simulink subsystem "GroundSystem"  (R2019b)
settings: Solver=VariableStepAuto  StartTime=0.0  StopTime=10.0  RelTol=1e-3
undefined symbols (not defined in the file): constr, Lbooth, loiterStates, params
libraries: simulink x4
settings Model: Creator=dylaneijkelhof  LastModifiedBy=dylaneijkelhof

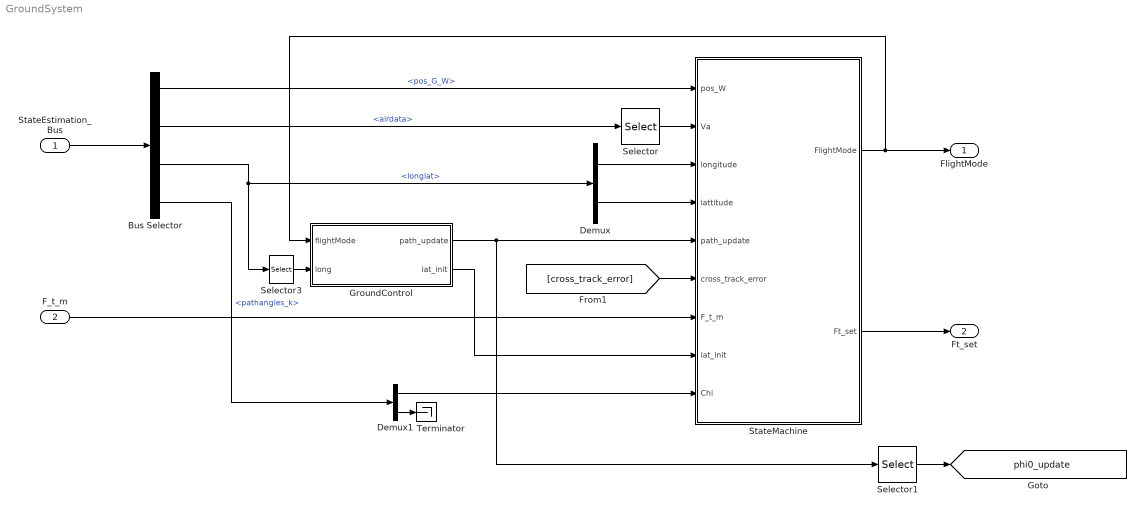
== system GroundSystem ==
  StateEstimation_Bus : Inport
  F_t_m : Inport  Port=2
  Bus Selector : BusSelector  OutputSignals=pos_G_W,airdata,longlat,pathangles_k
  Demux : Demux  Outputs=2
  Demux1 : Demux  Outputs=2
  GroundControl : Subsystem
  Selector : Selector  InputPortWidth=3  IndexOptions=Index vector (dialog)  Indices=1  OutputSizes=1
  Selector1 : Selector  InputPortWidth=3  IndexOptions=Index vector (dialog)  Indices=1  OutputSizes=1
  Selector3 : Selector  InputPortWidth=2  IndexOptions=Index vector (dialog)  Indices=1  OutputSizes=1
  StateMachine : Subsystem
  Terminator : Terminator
  FlightMode : Outport  VectorParamsAs1DForOutWhenUnconnected=off
  Ft_set : Outport  Port=2  VectorParamsAs1DForOutWhenUnconnected=off
  tag scope: phi0_update=global
  wires:
  Selector/1 -> StateMachine/2(Va)
  Bus Selector/2 -> Selector/1  "<airdata>"
  Bus Selector/1 -> StateMachine/1(pos_W)  "<pos_G_W>"
  StateEstimation_Bus/1 -> Bus Selector/1
  Demux/1 -> StateMachine/3(longitude)
  StateMachine/2(Ft_set) -> Ft_set/1
  Demux/2 -> StateMachine/4(lattitude)
  [cross_track_error] -> StateMachine/6(cross_track_error)
  F_t_m/1 -> StateMachine/7(F_t_m)
  Bus Selector/3 -> Demux/1, Selector3/1  "<longlat>"
  StateMachine/1(FlightMode) -> GroundControl/1(flightMode), FlightMode/1
  Selector1/1 -> [phi0_update]
  GroundControl/1(path_update) -> StateMachine/5(path_update), Selector1/1
  Selector3/1 -> GroundControl/2(long)
  GroundControl/2(lat_init) -> StateMachine/8(lat_init)
  Bus Selector/4 -> Demux1/1  "<pathangles_k>"
  Demux1/2 -> Terminator/1
  Demux1/1 -> StateMachine/9(Chi)

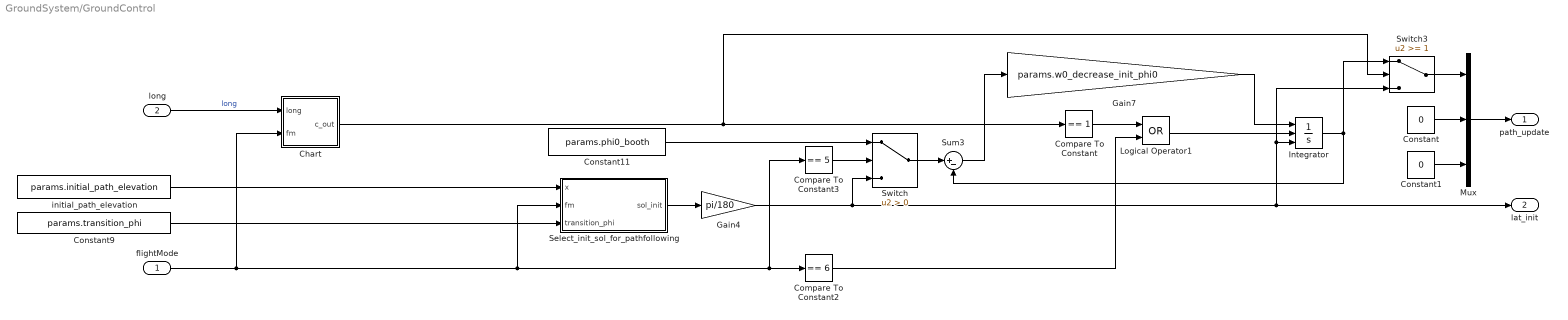
== system GroundSystem/GroundControl ==
  flightMode : Inport
  long : Inport  Port=2
  Chart : Stateflow chart  TreatAsAtomicUnit=on
  Compare To Constant : simulink/Logic and Bit Operations/Compare To Constant  relop===  const=1  OutDataTypeStr=boolean
  Compare To Constant2 : simulink/Logic and Bit Operations/Compare To Constant  relop===  const=6  OutDataTypeStr=boolean
  Compare To Constant3 : simulink/Logic and Bit Operations/Compare To Constant  relop===  const=5  OutDataTypeStr=boolean
  Constant : Constant  Value=0
  Constant1 : Constant  Value=0
  Constant11 : Constant  Value=params.phi0_booth
  Constant9 : Constant  Value=params.transition_phi
  Gain4 : Gain  Gain=pi/180
  Gain7 : Gain  Gain=params.w0_decrease_init_phi0
  Integrator : Integrator  ExternalReset=rising  InitialConditionSource=external
  Logical Operator1 : Logic  Operator=OR  AllPortsSameDT=off  OutDataTypeStr=boolean
  Mux : Mux  Inputs=3
  Select_init_sol_for_pathfollowing : Stateflow chart  TreatAsAtomicUnit=on
  Sum3 : Sum  Inputs=|+-
  Switch : Switch  Criteria=u2 > Threshold
  Switch3 : Switch  Threshold=1
  initial_path_elevation : Constant  Value=params.initial_path_elevation
  path_update : Outport  PortDimensions=[3,1]  VectorParamsAs1DForOutWhenUnconnected=off
  lat_init : Outport  Port=2  VectorParamsAs1DForOutWhenUnconnected=off
  wires:
  Constant11/1 -> Switch/1
  Constant9/1 -> Select_init_sol_for_pathfollowing/3(transition_phi)
  Switch3/1 -> Mux/1
  Gain7/1 -> Integrator/1
  Logical Operator1/1 -> Integrator/2
  Compare To Constant/1 -> Logical Operator1/1
  Integrator/1 -> Switch3/1, Sum3/2
  Gain4/1 -> Switch/3, lat_init/1, Integrator/3, Switch3/3
  Chart/1(c_out) -> Compare To Constant/1, Switch3/2
  long/1 -> Chart/1(long)  "long"
  initial_path_elevation/1 -> Select_init_sol_for_pathfollowing/1(x)
  Compare To Constant3/1 -> Switch/2
  Switch/1 -> Sum3/1
  Compare To Constant2/1 -> Logical Operator1/2
  flightMode/1 -> Chart/2(fm), Compare To Constant2/1, Compare To Constant3/1, Select_init_sol_for_pathfollowing/2(fm)
  Select_init_sol_for_pathfollowing/1(sol_init) -> Gain4/1
  Sum3/1 -> Gain7/1
  Mux/1 -> path_update/1
  Constant/1 -> Mux/2
  Constant1/1 -> Mux/3

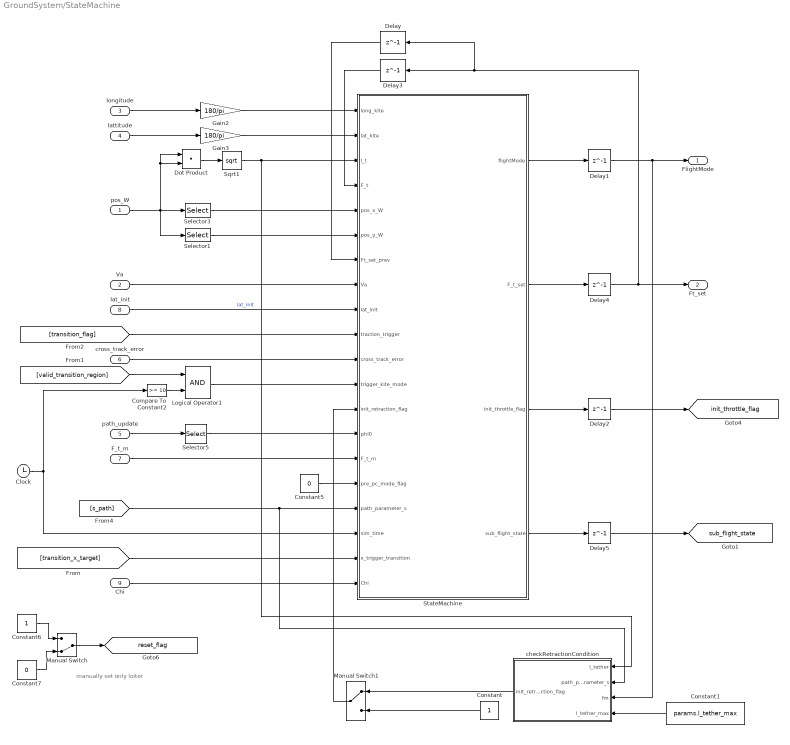
== system GroundSystem/StateMachine ==
  note: manually set only loiter
  pos_W : Inport
  Va : Inport  Port=2
  longitude : Inport  Port=3
  lattitude : Inport  Port=4
  path_update : Inport  Port=5
  cross_track_error : Inport  Port=6
  F_t_m : Inport  Port=7
  lat_init : Inport  Port=8
  Chi : Inport  Port=9
  Clock : Clock
  Compare To Constant2 : simulink/Logic and Bit Operations/Compare To Constant  relop=>=  const=10  OutDataTypeStr=boolean
  Constant : Constant
  Constant1 : Constant  Value=params.l_tether_max
  Constant5 : Constant  Value=0
  Constant6 : Constant
  Constant7 : Constant  Value=0
  Delay : Delay  DelayLength=1  InitialCondition=100
  Delay1 : Delay  DelayLength=1
  Delay2 : Delay  DelayLength=1  InitialCondition=1
  Delay3 : Delay  DelayLength=1  InitialCondition=100
  Delay4 : Delay  DelayLength=1
  Delay5 : Delay  DelayLength=1  InitialCondition=1
  Dot Product : DotProduct  InputSameDT=on  OutDataTypeStr=Inherit: Inherit via internal rule
  Gain2 : Gain  Gain=180/pi
  Gain3 : Gain  Gain=180/pi
  Logical Operator1 : Logic  AllPortsSameDT=off  OutDataTypeStr=boolean
  Manual Switch : ManualSwitch  CurrentSetting=0
  Manual Switch1 : ManualSwitch
  Selector1 : Selector  InputPortWidth=3  IndexOptions=Index vector (dialog)  Indices=2  OutputSizes=1
  Selector3 : Selector  InputPortWidth=3  IndexOptions=Index vector (dialog)  Indices=1  OutputSizes=1
  Selector5 : Selector  InputPortWidth=3  IndexOptions=Index vector (dialog)  Indices=1  OutputSizes=1
  Sqrt1 : Sqrt  SaturateOnIntegerOverflow=on
  StateMachine : Stateflow chart  TreatAsAtomicUnit=on  mask{F_T_traction_set=params.F_t_traction_set, F_set_retraction=params.F_t_retraction_set*params.F_t_traction_set, l_t_min=params.l_tether_min, l_t_max=params.l_tether_max, a_booth=params.a_booth, b_booth=params.b_booth, lat_trans=0, alpha2=params.ft_smooth_2, crosstrackerror_condition=params.crosstrackerror_condition, Vamin=constr.Va_min, Ft_set_loiter=loiterStates.Ft_set_loiter}
      mask prompts: F_T_traction_set "Traction force"; F_set_retraction "Retraction force"; l_t_min "Min. tether length"; l_t_max "Max. tether length"; a_booth "abooth"; b_booth "bbooth"; alpha2 "interpolation factor retrac 2 trac"
  checkRetractionCondition : Stateflow chart  TreatAsAtomicUnit=on
  FlightMode : Outport  VectorParamsAs1DForOutWhenUnconnected=off
  Ft_set : Outport  Port=2  VectorParamsAs1DForOutWhenUnconnected=off
  tag scope: init_throttle_flag=global, reset_flag=global, sub_flight_state=global
  wires:
  Chi/1 -> StateMachine/20(Chi)
  [transition_x_target] -> StateMachine/19(x_trigger_transition)
  Delay5/1 -> [sub_flight_state]
  Constant/1 -> Manual Switch1/2
  checkRetractionCondition/1(init_retraction_flag) -> Manual Switch1/1
  lat_init/1 -> StateMachine/9(lat_init)  "lat_init"
  [s_path] -> StateMachine/17(path_parameter_s), checkRetractionCondition/2(path_parameter_s)
  Clock/1 -> StateMachine/18(sim_time), Compare To Constant2/1
  Manual Switch/1 -> [reset_flag]
  Constant7/1 -> Manual Switch/2
  Constant6/1 -> Manual Switch/1
  [transition_flag] -> StateMachine/10(traction_trigger)
  Constant5/1 -> StateMachine/16(pre_pc_mode_flag)
  F_t_m/1 -> StateMachine/15(F_t_m)
  StateMachine/4(sub_flight_state) -> Delay5/1
  Delay4/1 -> Delay3/1, Delay/1, Ft_set/1
  Sqrt1/1 -> StateMachine/3(l_t), checkRetractionCondition/1(l_tether)
  Gain3/1 -> StateMachine/2(lat_kite)
  path_update/1 -> Selector5/1
  Selector5/1 -> StateMachine/14(phi0)
  Delay3/1 -> StateMachine/4(F_t)
  StateMachine/1(flightMode) -> Delay1/1
  Gain2/1 -> StateMachine/1(long_kite)
  pos_W/1 -> Selector3/1, Selector1/1, Dot Product/2, Dot Product/1
  Selector3/1 -> StateMachine/5(pos_x_W)
  Dot Product/1 -> Sqrt1/1
  Delay/1 -> StateMachine/7(Ft_set_prev)
  Selector1/1 -> StateMachine/6(pos_y_W)
  cross_track_error/1 -> StateMachine/11(cross_track_error)
  Logical Operator1/1 -> StateMachine/12(trigger_kite_mode)
  Compare To Constant2/1 -> Logical Operator1/2
  [valid_transition_region] -> Logical Operator1/1
  Delay1/1 -> checkRetractionCondition/3(fm), FlightMode/1
  StateMachine/3(init_throttle_flag) -> Delay2/1
  Delay2/1 -> [init_throttle_flag]
  longitude/1 -> Gain2/1
  lattitude/1 -> Gain3/1
  StateMachine/2(F_t_set) -> Delay4/1
  Va/1 -> StateMachine/8(Va)
  Constant1/1 -> checkRetractionCondition/4(l_tether_max)
  Manual Switch1/1 -> StateMachine/13(init_retraction_flag)

== stateflow chart GroundSystem/StateMachine/StateMachine ==
  state loiter
    entry: flightMode = 1;
    during: F_t_set = Ft_set_loiter;
    entry: init_throttle_flag = 1;
    entry: sub_flight_state = 1;
  state Traction4 % slowly increase tether force
    entry: flightMode=5;
    during: F_t_set = calcSetpoint(alpha2,Ft_set_prev,Ft_set_loiter);
    exit: init_throttle_flag = 1;
    entry: sub_flight_state = 2;
  note: F_t_m>F_set_retraction
  note: pos_x_W<x_trigger_transition
  state Retraction3 [commented out]
    entry: flightMode=6;
    entry: F_t_set =calcSetpoint(1,Ft_set_prev,3000);
    %entry: F_t_set = 0;
    entry: reelin_flag = 1;
    entry: sub_flight_state = 8;
    entry: path_captured_flag = 0;
  state Traction2 % slowly increase tether force
    entry: flightMode=5;
    during: F_t_set = calcSetpoint(alpha2,Ft_set_prev,F_T_traction_set);
    exit: init_throttle_flag = 1;
    entry: sub_flight_state = 2;
  state Retraction1
    entry: flightMode=6;
    entry: F_t_set =calcSetpoint(alpha2,F_set_retraction,Ft_set_prev);
    entry: reelin_flag = 1;
    entry: sub_flight_state = 7;
    entry: path_captured_flag = 0;
  state Retraction
    entry: flightMode=6;
    entry: reelin_flag = 1;
    during: F_t_set = calcSetpoint(alpha2,F_set_retraction,Ft_set_prev);
    entry: sub_flight_state = 6;
  state Traction1
    entry: flightMode=5;
    during: F_t_set = calcSetpoint(alpha2,Ft_set_prev,F_T_traction_set);
    entry: sub_flight_state = 3;
  state Traction3
    entry: flightMode=5;
    entry: path_captured_flag = 1;
    entry: init_throttle_flag = 0;
    during: F_t_set = calcSetpoint(alpha2,Ft_set_prev,F_T_traction_set);
    entry: sub_flight_state = 4;
  state Trans2Retract
    entry: flightMode=5;
    during: F_t_set = calcSetpoint(alpha2,Ft_set_prev,F_T_traction_set);
    entry: sub_flight_state = 5;
  (default) -> loiter
  loiter -> Traction4 % slowly increase tether force : [trigger_kite_mode == 1]
  Traction4 % slowly increase tether force -> Traction2 % slowly increase tether force : [pre_pc_mode_flag==0]
  Retraction1 -> Retraction3 [commented out] : [x_trigger_transition>0]
  Retraction1 -> Traction1 : [pos_x_W<x_trigger_transition]
  Traction2 % slowly increase tether force -> Traction3 : [long_kite>0]
  Retraction -> Retraction1 : [F_t_m<1.1*F_set_retraction]
  (junction 286) -> Retraction
  Traction1 -> Traction3 : [cross_track_error < crosstrackerror_condition&&Va>=Vamin]
  Traction3 -> Trans2Retract : [(l_t>l_t_max||init_retraction_flag)]
  Traction3 -> Trans2Retract [commented out] : [(l_t>l_t_max||init_retraction_flag)&& (path_parameter_s >= (5*pi/3+.5*pi/180) && path_parameter_s <=5*pi/3+1*pi/180)]
  Traction3 -> Trans2Retract [commented out] : [(l_t>l_t_max||init_retraction_flag)&& (path_parameter_s >= (2*pi/3+.5*pi/180) && path_parameter_s <= 2*pi/3+1*pi/180)]
  Trans2Retract -> (junction 286) [order 1] : [path_parameter_s >= (pi/2+.5*pi/180) && path_parameter_s <= pi/2+1*pi/180]
  (junction 319) -> (junction 286)
  Trans2Retract -> (junction 319) [order 2] : [path_parameter_s >= (3*pi/2+.5*pi/180) && path_parameter_s <=3*pi/2+1*pi/180]
  (junction 348) -> (junction 319) [commented out]
  Trans2Retract -> (junction 348) [commented out] : [Chi >= (0-0.5*pi/180) && Chi <= 0+0.5*pi/180]
  data: Ft_set function_output; alpha1_ function_input; Ft_set_prev_ function_input; F_T_traction_set_ function_input; flightMode output; long_kite input; lat_kite input; l_t input; F_t input; Lbooth parameter; pos_x_W input; pos_y_W input; F_t_set output; F_T_traction_set parameter double; F_set_retraction parameter; a_booth parameter; b_booth parameter; l_t_min parameter; lat_trans parameter; l_t_max parameter; Ft_set_prev input; alpha2 parameter; Va input; lat_init input; traction_trigger input; cross_track_error input; trigger_kite_mode input; init_throttle_flag output size=1; crosstrackerror_condition parameter; Vamin parameter; init_retraction_flag input; Ft_set_loiter parameter; phi0 input; F_t_m input; sub_flight_state output =1; pre_pc_mode_flag input; path_parameter_s input; sim_time input; reelin_flag local; path_captured_flag local; x_trigger_transition input; side local; Chi input
  function Ft_set = calcSetpoint(alpha1_,Ft_set_prev_, F_T_traction_set_):
    | % Copyright 2020 Delft University of Technology
    | %
    | % Licensed under the Apache License, Version 2.0 (the "License");
    | % you may not use this file except in compliance with the License.
    | % You may obtain a copy of the License at
    | %
    | %      http://www.apache.org/licenses/LICENSE-2.0
    | %
    | % Unless required by applicable law or agreed to in writing, software
    | % distributed under the License is distributed on an "AS IS" BASIS,
    | % WITHOUT WARRANTIES OR CONDITIONS OF ANY KIND, either express or implied.
    | % See the License for the specific language governing permissions and
    | % limitations under the License. 
    | 
    | function Ft_set = calcSetpoint(alpha1_,Ft_set_prev_, F_T_traction_set_)
    |  
    | Ft_set =  alpha1_ * F_T_traction_set_ +(1-alpha1_)*Ft_set_prev_;
    | 
    | end

== stateflow chart GroundSystem/StateMachine/checkRetractionCondition ==
  state calcIncrement1
    during: l_tether_predict =l_tether+l_tether-l0;
  state init2
    entry: init_retraction_flag=1;
  state init
    entry: init_retraction_flag=0;
  state calcIncrement
    during: l_tether_predict =l_tether+l_tether-l0;
  state set0length
    entry: l0 = l_tether;
  calcIncrement1 -> (junction 38) : [path_parameter_s >= (3*pi/2-1*pi/180) && path_parameter_s <=3*pi/2+1*pi/180 ]
  init2 -> init : [fm==6]
  (junction 38) -> init2 [order 1] : [l_tether_predict>=l_tether_max*1.15]
  set0length -> calcIncrement1 [order 4] : [path_parameter_s >= (pi/2-1*pi/180) && path_parameter_s <= pi/2+1*pi/180]
  (default) -> init
  set0length -> init [order 2] : [fm==6]
  (junction 38) -> set0length [order 2]
  calcIncrement -> (junction 38) : [path_parameter_s >= (pi/2-1*pi/180) && path_parameter_s <= pi/2+1*pi/180]
  set0length -> init [order 3] : [fm==6]
  init -> set0length : [path_parameter_s >= (pi/2-1*pi/180) && path_parameter_s <= pi/2+1*pi/180 &&fm==5]
  set0length -> calcIncrement [order 1] : [path_parameter_s >= (3*pi/2-1*pi/180) && path_parameter_s <=3*pi/2+1*pi/180 ]
  data: l_tether input; path_parameter_s input; fm input; l0 local; init_retraction_flag output; l_tether_max input; dl local; l_tether_predict local

== stateflow chart GroundSystem/GroundControl/Chart ==
  note: Counter structure that counts the figures of 8
      | during the traction phase and resets as soon as
      | the retraction phase is triggered
  state counter1
    entry: c=c+1;
    entry: c_out = c;
  state counter2
    entry: c=c+1;
    entry: c_out = c;
  state s1
  state init
    entry:c=-1;
    entry: c_out = c;
  state reset
    entry: c=-1;
    entry: c_out = c;
  state counter3
    entry: c=c+1;
    entry: c_out = c;
  state s4
  state counter
    entry: c=c+1;
    entry: c_out = c;
  reset -> s1 [order 1] : [long>0]
  counter1 -> reset [order 1] : [fm==6]
  counter1 -> counter2 [order 2] : [long<0]
  counter2 -> counter1 [order 1] : [long>0]
  s1 -> counter2 : [long<0]
  init -> s1 [order 1] : [long>0]
  counter2 -> reset [order 2] : [fm==6]
  (default) -> init
  reset -> s4 [order 2] : [long<=0]
  counter3 -> reset [order 1] : [fm==6]
  counter -> reset [order 2] : [fm==6]
  init -> s4 [order 2] : [long<=0]
  s4 -> counter3 : [long>0]
  counter -> counter3 [order 1] : [long>0]
  counter3 -> counter [order 2] : [long<0]
  data: long input; fm input; c_out output; c local

== stateflow chart GroundSystem/GroundControl/Select_init_sol_for_pathfollowing ==
  state Init
    entry: sol_init = x;
  state Pumping
    entry: sol_init = transition_phi;
  (default) -> Init
  Init -> Pumping : [fm == 6]
  data: x input; fm input; sol_init output; transition_phi input
